simulink model "Calculator"  (R2021a)
settings: Solver=VariableStepAuto  StartTime=0.0  StopTime=10.0  RelTol=1e-3
settings Model: Creator=Moamen_Hamed  LastModifiedBy=Moamen_Hamed

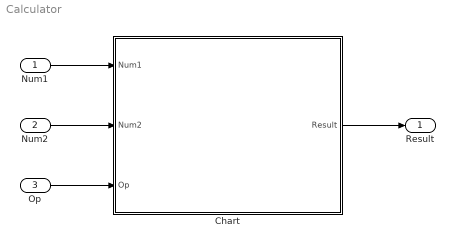
== system Calculator ==
  Num1 : Inport
  Num2 : Inport  Port=2
  Op : Inport  Port=3
  Chart : Stateflow chart  TreatAsAtomicUnit=on
  Result : Outport
  wires:
  Num1/1 -> Chart/1(Num1)
  Num2/1 -> Chart/2(Num2)
  Op/1 -> Chart/3(Op)
  Chart/1(Result) -> Result/1

== stateflow chart Calculator/Chart ==
  state Add(Num1,Num2) [function]
    (default) -> (junction 2) : {Result = Num1+Num2;}
  state Calculator
    (default) -> (junction 48)
    (junction 48) -> (junction 49) [order 1] : [Op == 0]
    (junction 48) -> (junction 50) [order 2]
    (junction 49) -> (junction 57) : {Add(Num1,Num2);}
    (junction 50) -> (junction 51) [order 1] : [Op == 1]
    (junction 50) -> (junction 52) [order 2]
    (junction 51) -> (junction 56) : {Sub(Num1,Num2);}
    (junction 52) -> (junction 53) [order 1] : [Op == 2]
    (junction 52) -> (junction 54) [order 2] : {Div(Num1,Num2);}
    (junction 53) -> (junction 55) : {Mul(Num1,Num2);}
    (junction 55) -> (junction 54)
    (junction 56) -> (junction 55)
    (junction 57) -> (junction 56)
    (junction 54) -> (junction 58)
  state Sub(Num1,Num2) [function]
    (default) -> (junction 5) : {Result=Num1-Num2;}
  state Mul(Num1,Num2) [function]
    (default) -> (junction 8) : {Result=Num1*Num2;}
  state Div(Num1,Num2) [function]
    (default) -> (junction 25)
    (junction 25) -> (junction 26) [order 1] : [Num2==0]
    (junction 25) -> (junction 27) [order 2] : {Result=Num1/Num2;}
    (junction 26) -> (junction 28) : {Result=-1;}
    (junction 28) -> (junction 27)
    (junction 27) -> (junction 29)
  (default) -> Calculator
  data: Num1 function_input; Num2 function_input; Num1 function_input; Num2 function_input; Num1 function_input; Num2 function_input; Num1 function_input; Num2 function_input; Num1 input; Num2 input; Op input; Result output
